simulink model "x2_Robot_Kin"  (R2024b)
settings: Solver=VariableStepAuto  StartTime=0.0  StopTime=inf  RelTol=1e-3  EnableMultiTasking=on
libraries: vrlib x7, simulink x6
settings Model: Creator=jorgemartins  LastModifiedBy=pinto
settings SolverCC: AlgebraicLoopSolver=TrustRegion
settings DataIOCC: LimitDataPoints=on  ReturnWorkspaceOutputs=off
settings OptimizationCC: LifeSpan=inf
settings DebuggingCC: UnconnectedInputMsg=warning  UnconnectedOutputMsg=warning  UnconnectedLineMsg=warning  AllowSymbolicDim=off  SFUnexpectedBacktrackingDiag=warning  SFNoUnconditionalDefaultTransitionDiag=warning  SFExecutionAtInitializationDiag=none  ArithmeticOperatorsInVariantConditions=warning
settings ModelReferenceCC: EnableRefExpFcnMdlSchedulingChecks=on  PropagateSignalLabelsOutOfModel=off
settings SFSimCC: SimUseLocalCustomCode=off  CustomCodeUndefinedFunction=UseInterfaceOnly
settings RTWCC: RTWUseLocalCustomCode=off  GPUComputeCapability=3.5
settings CodeAppCC: StateflowObjectComments=on
settings GRTTargetCC: TargetLangStandard=C89/C90 (ANSI)
settings ConfigComp: CovMetricSettings=dw  CovSaveCumulativeToWorkspaceVar=on  CovSaveSingleToWorkspaceVar=on  CovExternalEMLEnable=off

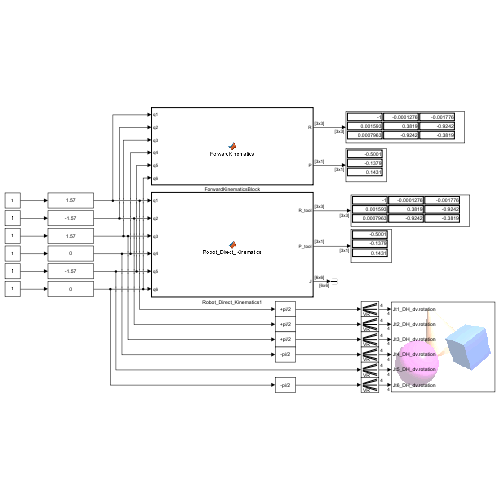
[thumbnail: Simulink's stored preview of the top-level diagram]
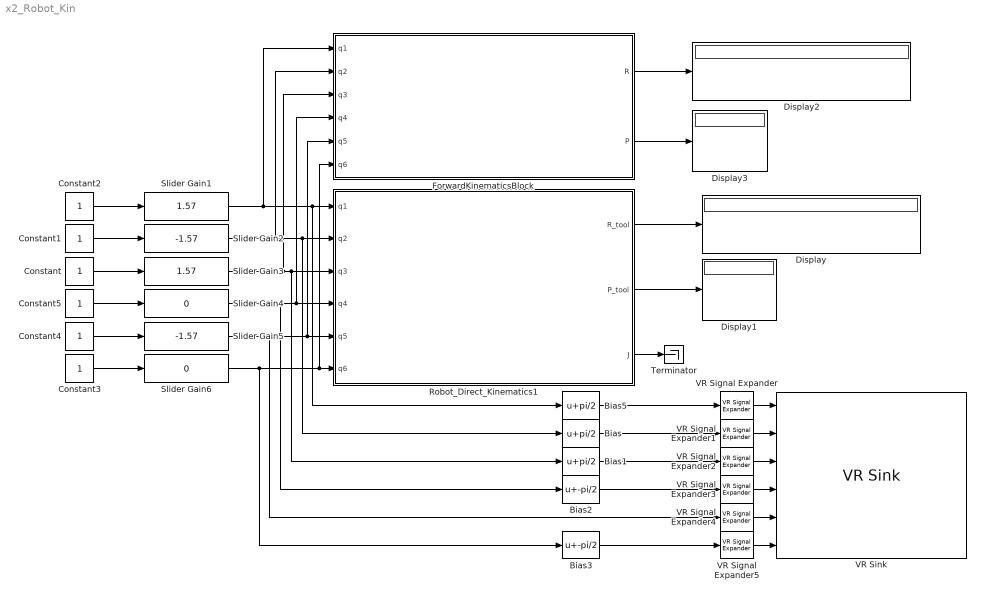
== system x2_Robot_Kin ==
  Bias : Bias  Bias=pi/2  SaturateOnIntegerOverflow=off
  Bias1 : Bias  Bias=pi/2  SaturateOnIntegerOverflow=off
  Bias2 : Bias  Bias=-pi/2  SaturateOnIntegerOverflow=off
  Bias3 : Bias  Bias=-pi/2  SaturateOnIntegerOverflow=off
  Bias5 : Bias  Bias=pi/2  SaturateOnIntegerOverflow=off
  Constant{,1..5} (6 alike) : Constant
  Display{,1..3} (4 alike) : Display
  ForwardKinematicsBlock : MATLAB Function  TreatAsAtomicUnit=on
  Robot_Direct_Kinematics1 : MATLAB Function  TreatAsAtomicUnit=on
  Slider Gain1 : simulink/Math Operations/Slider Gain  gain=1.57  low=-3.14  high=3.14
  Slider Gain2 : simulink/Math Operations/Slider Gain  gain=-1.57  low=-3.14  high=3.14
  Slider Gain3 : simulink/Math Operations/Slider Gain  gain=1.57  low=-3.14  high=3.14
  Slider Gain4 : simulink/Math Operations/Slider Gain  gain=0  low=-3.14  high=3.14
  Slider Gain5 : simulink/Math Operations/Slider Gain  gain=-1.57  low=-3.14  high=3.14
  Slider Gain6 : simulink/Math Operations/Slider Gain  gain=0  low=-3.14  high=3.14
  Terminator : Terminator
  VR Signal Expander{,1..5} (6 alike) : vrlib/VR Signal Expander  outwidth=4  outidx=[4]
  VR Sink : vrlib/VR Sink  InstantiateOnLoad=on  SampleTime=0.1  ViewEnable=on  RemoteChange=off  RemoteView=off  FieldsWritten=Jt1_DH_dv.rotation.4.1.1.double#Jt2_DH_dv.rotation.4.1.1.double#Jt3_DH_dv.rotation.4.1.1.double#Jt4_DH_dv.rotation.4.1.1.double#Jt5_DH_dv.rotation.4.1.1.double#Jt6_DH_dv.rotation.4.1.1.double  WorldFileName=vrrobot.wrl  WorldDescription=D-H Reference Frames for Virtual Reality Robot  AutoView=off  VideoDimensions=[]  AllowVariableSize=off
  wires:
  Robot_Direct_Kinematics1/1(R_tool) -> Display/1
  Robot_Direct_Kinematics1/2(P_tool) -> Display1/1
  Constant/1 -> Slider Gain3/1
  Slider Gain3/1 -> ForwardKinematicsBlock/3(q3), Robot_Direct_Kinematics1/3(q3), Bias1/1
  Constant2/1 -> Slider Gain1/1
  Slider Gain1/1 -> ForwardKinematicsBlock/1(q1), Robot_Direct_Kinematics1/1(q1), Bias5/1
  Constant1/1 -> Slider Gain2/1
  Slider Gain2/1 -> ForwardKinematicsBlock/2(q2), Robot_Direct_Kinematics1/2(q2), Bias/1
  Bias/1 -> VR Signal Expander1/1
  Bias1/1 -> VR Signal Expander2/1
  Constant4/1 -> Slider Gain5/1
  Slider Gain6/1 -> Robot_Direct_Kinematics1/6(q6), ForwardKinematicsBlock/6(q6), Bias3/1
  Constant3/1 -> Slider Gain6/1
  Slider Gain4/1 -> Robot_Direct_Kinematics1/4(q4), ForwardKinematicsBlock/4(q4), Bias2/1
  Constant5/1 -> Slider Gain4/1
  Bias3/1 -> VR Signal Expander5/1
  Slider Gain5/1 -> Robot_Direct_Kinematics1/5(q5), ForwardKinematicsBlock/5(q5), VR Signal Expander4/1
  Bias2/1 -> VR Signal Expander3/1
  Bias5/1 -> VR Signal Expander/1
  VR Signal Expander/1 -> VR Sink/1
  VR Signal Expander1/1 -> VR Sink/2
  VR Signal Expander2/1 -> VR Sink/3
  VR Signal Expander3/1 -> VR Sink/4
  VR Signal Expander4/1 -> VR Sink/5
  VR Signal Expander5/1 -> VR Sink/6
  ForwardKinematicsBlock/2(P) -> Display3/1
  ForwardKinematicsBlock/1(R) -> Display2/1
  Robot_Direct_Kinematics1/3(J) -> Terminator/1

== matlab function x2_Robot_Kin/ForwardKinematicsBlock ==
  data: q1 input; R output; q2 input; q3 input; q4 input; q5 input; q6 input; P output
function [R, P] = ForwardKinematics(q1, q2, q3, q4, q5, q6)

DH = [ 0     q1  0     pi/2      pi/2;
       0     q2  0    -pi/2      pi/2;
       0.4   q3  0     pi/2      pi/2;
       0     q4  0.1   pi/2     -pi/2;
       0.5   q5  0    -pi/2      0;
       0.1   q6  0     pi/2-pi/8 -pi/2;
       0.15  0   0     0         0 ];

T = eye(4);

for i = 1:size(DH,1)
    d = DH(i,1);
    theta = DH(i,2) + DH(i,5);
    a = DH(i,3);
    alpha = DH(i,4);

    A = [ cos(theta), -sin(theta)*cos(alpha),  sin(theta)*sin(alpha), a*cos(theta);
          sin(theta),  cos(theta)*cos(alpha), -cos(theta)*sin(alpha), a*sin(theta);
          0,           sin(alpha),             cos(alpha),            d;
          0,           0,                      0,                     1 ];

    T = T * A;
end

R = T(1:3, 1:3);
P = T(1:3, 4);

== matlab function x2_Robot_Kin/Robot_Direct_Kinematics1 ==
  data: q1 input; R_tool output; q2 input; q3 input; q4 input; q5 input; q6 input; P_tool output; J output
function [R_tool,P_tool,J] = Robot_Direct_Kinematics(q1,q2,q3,q4,q5,q6)
%#codegen

%    This function was generated by the Symbolic Math Toolbox version 24.2.
%    22-May-2025 17:53:28

% q1 = complex(q1);  % if required to enforce complex operations
% q2 = complex(q2);  % if required to enforce complex operations
% q3 = complex(q3);  % if required to enforce complex operations
% q4 = complex(q4);  % if required to enforce complex operations
% q5 = complex(q5);  % if required to enforce complex operations
% q6 = complex(q6);  % if required to enforce complex operations
et1 = cos(q5).*sin(q1).*sin(q3).*sqrt(sqrt(2.0)+2.0).*(-1.0./2.0)-(cos(q1).*cos(q2).*sin(q4).*sin(q6).*sqrt(-sqrt(2.0)+2.0))./2.0-(cos(q3).*cos(q4).*sin(q1).*sin(q6).*sqrt(-sqrt(2.0)+2.0))./2.0-(cos(q6).*sin(q1).*sin(q3).*sin(q5).*sqrt(-sqrt(2.0)+2.0))./2.0-(cos(q1).*cos(q3).*cos(q5).*sin(q2).*sqrt(sqrt(2.0)+2.0))./2.0-(cos(q1).*cos(q2).*cos(q4).*sin(q5).*sqrt(sqrt(2.0)+2.0))./2.0+(cos(q3).*sin(q1).*sin(q4).*sin(q5).*sqrt(sqrt(2.0)+2.0))./2.0;
et2 = (cos(q1).*cos(q2).*cos(q4).*cos(q5).*cos(q6).*sqrt(-sqrt(2.0)+2.0))./2.0-(cos(q1).*cos(q3).*cos(q6).*sin(q2).*sin(q5).*sqrt(-sqrt(2.0)+2.0))./2.0-(cos(q3).*cos(q5).*cos(q6).*sin(q1).*sin(q4).*sqrt(-sqrt(2.0)+2.0))./2.0+(cos(q1).*cos(q4).*sin(q2).*sin(q3).*sin(q6).*sqrt(-sqrt(2.0)+2.0))./2.0-(cos(q1).*sin(q2).*sin(q3).*sin(q4).*sin(q5).*sqrt(sqrt(2.0)+2.0))./2.0+(cos(q1).*cos(q5).*cos(q6).*sin(q2).*sin(q3).*sin(q4).*sqrt(-sqrt(2.0)+2.0))./2.0;
et3 = cos(q1).*cos(q5).*sin(q3).*sqrt(sqrt(2.0)+2.0).*(-1.0./2.0)-(cos(q1).*cos(q3).*cos(q4).*sin(q6).*sqrt(-sqrt(2.0)+2.0))./2.0-(cos(q1).*cos(q6).*sin(q3).*sin(q5).*sqrt(-sqrt(2.0)+2.0))./2.0+(cos(q2).*sin(q1).*sin(q4).*sin(q6).*sqrt(-sqrt(2.0)+2.0))./2.0+(cos(q3).*cos(q5).*sin(q1).*sin(q2).*sqrt(sqrt(2.0)+2.0))./2.0+(cos(q2).*cos(q4).*sin(q1).*sin(q5).*sqrt(sqrt(2.0)+2.0))./2.0+(cos(q1).*cos(q3).*sin(q4).*sin(q5).*sqrt(sqrt(2.0)+2.0))./2.0-(cos(q2).*cos(q4).*cos(q5).*cos(q6).*sin(q1).*sqrt(-sqrt(2.0)+2.0))./2.0;
et4 = cos(q1).*cos(q3).*cos(q5).*cos(q6).*sin(q4).*sqrt(-sqrt(2.0)+2.0).*(-1.0./2.0)+(cos(q3).*cos(q6).*sin(q1).*sin(q2).*sin(q5).*sqrt(-sqrt(2.0)+2.0))./2.0-(cos(q4).*sin(q1).*sin(q2).*sin(q3).*sin(q6).*sqrt(-sqrt(2.0)+2.0))./2.0+(sin(q1).*sin(q2).*sin(q3).*sin(q4).*sin(q5).*sqrt(sqrt(2.0)+2.0))./2.0-(cos(q5).*cos(q6).*sin(q1).*sin(q2).*sin(q3).*sin(q4).*sqrt(-sqrt(2.0)+2.0))./2.0;
et5 = cos(q5).*sin(q1).*sin(q3).*sqrt(-sqrt(2.0)+2.0).*(-1.0./2.0)-(cos(q1).*cos(q3).*cos(q5).*sin(q2).*sqrt(-sqrt(2.0)+2.0))./2.0-(cos(q1).*cos(q2).*cos(q4).*sin(q5).*sqrt(-sqrt(2.0)+2.0))./2.0+(cos(q3).*sin(q1).*sin(q4).*sin(q5).*sqrt(-sqrt(2.0)+2.0))./2.0+(cos(q1).*cos(q2).*sin(q4).*sin(q6).*sqrt(sqrt(2.0)+2.0))./2.0+(cos(q3).*cos(q4).*sin(q1).*sin(q6).*sqrt(sqrt(2.0)+2.0))./2.0+(cos(q6).*sin(q1).*sin(q3).*sin(q5).*sqrt(sqrt(2.0)+2.0))./2.0;
et6 = cos(q1).*sin(q2).*sin(q3).*sin(q4).*sin(q5).*sqrt(-sqrt(2.0)+2.0).*(-1.0./2.0)-(cos(q1).*cos(q2).*cos(q4).*cos(q5).*cos(q6).*sqrt(sqrt(2.0)+2.0))./2.0+(cos(q1).*cos(q3).*cos(q6).*sin(q2).*sin(q5).*sqrt(sqrt(2.0)+2.0))./2.0+(cos(q3).*cos(q5).*cos(q6).*sin(q1).*sin(q4).*sqrt(sqrt(2.0)+2.0))./2.0-(cos(q1).*cos(q4).*sin(q2).*sin(q3).*sin(q6).*sqrt(sqrt(2.0)+2.0))./2.0-(cos(q1).*cos(q5).*cos(q6).*sin(q2).*sin(q3).*sin(q4).*sqrt(sqrt(2.0)+2.0))./2.0;
et7 = cos(q1).*cos(q5).*sin(q3).*sqrt(-sqrt(2.0)+2.0).*(-1.0./2.0)+(cos(q3).*cos(q5).*sin(q1).*sin(q2).*sqrt(-sqrt(2.0)+2.0))./2.0+(cos(q2).*cos(q4).*sin(q1).*sin(q5).*sqrt(-sqrt(2.0)+2.0))./2.0+(cos(q1).*cos(q3).*sin(q4).*sin(q5).*sqrt(-sqrt(2.0)+2.0))./2.0+(cos(q1).*cos(q3).*cos(q4).*sin(q6).*sqrt(sqrt(2.0)+2.0))./2.0+(cos(q1).*cos(q6).*sin(q3).*sin(q5).*sqrt(sqrt(2.0)+2.0))./2.0-(cos(q2).*sin(q1).*sin(q4).*sin(q6).*sqrt(sqrt(2.0)+2.0))./2.0;
et8 = (sin(q1).*sin(q2).*sin(q3).*sin(q4).*sin(q5).*sqrt(-sqrt(2.0)+2.0))./2.0+(cos(q2).*cos(q4).*cos(q5).*cos(q6).*sin(q1).*sqrt(sqrt(2.0)+2.0))./2.0+(cos(q1).*cos(q3).*cos(q5).*cos(q6).*sin(q4).*sqrt(sqrt(2.0)+2.0))./2.0-(cos(q3).*cos(q6).*sin(q1).*sin(q2).*sin(q5).*sqrt(sqrt(2.0)+2.0))./2.0+(cos(q4).*sin(q1).*sin(q2).*sin(q3).*sin(q6).*sqrt(sqrt(2.0)+2.0))./2.0+(cos(q5).*cos(q6).*sin(q1).*sin(q2).*sin(q3).*sin(q4).*sqrt(sqrt(2.0)+2.0))./2.0;
mt1 = [cos(q1).*cos(q3).*cos(q4).*cos(q6)-cos(q2).*cos(q6).*sin(q1).*sin(q4)-cos(q1).*sin(q3).*sin(q5).*sin(q6)-cos(q2).*cos(q4).*cos(q5).*sin(q1).*sin(q6)-cos(q1).*cos(q3).*cos(q5).*sin(q4).*sin(q6)+cos(q4).*cos(q6).*sin(q1).*sin(q2).*sin(q3)+cos(q3).*sin(q1).*sin(q2).*sin(q5).*sin(q6)-cos(q5).*sin(q1).*sin(q2).*sin(q3).*sin(q4).*sin(q6),cos(q1).*cos(q2).*cos(q6).*sin(q4)+cos(q3).*cos(q4).*cos(q6).*sin(q1)-sin(q1).*sin(q3).*sin(q5).*sin(q6)+cos(q1).*cos(q2).*cos(q4).*cos(q5).*sin(q6)-cos(q1).*cos(q4).*cos(q6).*sin(q2).*sin(q3)-cos(q1).*cos(q3).*sin(q2).*sin(q5).*sin(q6)-cos(q3).*cos(q5).*sin(q1).*sin(q4).*sin(q6)+cos(q1).*cos(q5).*sin(q2).*sin(q3).*sin(q4).*sin(q6)];
mt2 = [cos(q6).*sin(q2).*sin(q4)+cos(q2).*cos(q4).*cos(q6).*sin(q3)+cos(q2).*cos(q3).*sin(q5).*sin(q6)+cos(q4).*cos(q5).*sin(q2).*sin(q6)-cos(q2).*cos(q5).*sin(q3).*sin(q4).*sin(q6),et3+et4,et1+et2];
mt3 = [cos(q4).*sin(q2).*sin(q5).*sqrt(sqrt(2.0)+2.0).*(-1.0./2.0)-(sin(q2).*sin(q4).*sin(q6).*sqrt(-sqrt(2.0)+2.0))./2.0+(cos(q2).*cos(q3).*cos(q5).*sqrt(sqrt(2.0)+2.0))./2.0+(cos(q2).*cos(q3).*cos(q6).*sin(q5).*sqrt(-sqrt(2.0)+2.0))./2.0+(cos(q4).*cos(q5).*cos(q6).*sin(q2).*sqrt(-sqrt(2.0)+2.0))./2.0-(cos(q2).*cos(q4).*sin(q3).*sin(q6).*sqrt(-sqrt(2.0)+2.0))./2.0+(cos(q2).*sin(q3).*sin(q4).*sin(q5).*sqrt(sqrt(2.0)+2.0))./2.0-(cos(q2).*cos(q5).*cos(q6).*sin(q3).*sin(q4).*sqrt(-sqrt(2.0)+2.0))./2.0];
mt4 = [et7+et8,et5+et6,(sin(q2).*sin(q4).*sin(q6).*sqrt(sqrt(2.0)+2.0))./2.0+(cos(q2).*cos(q3).*cos(q5).*sqrt(-sqrt(2.0)+2.0))./2.0-(cos(q4).*sin(q2).*sin(q5).*sqrt(-sqrt(2.0)+2.0))./2.0+(cos(q2).*sin(q3).*sin(q4).*sin(q5).*sqrt(-sqrt(2.0)+2.0))./2.0-(cos(q2).*cos(q3).*cos(q6).*sin(q5).*sqrt(sqrt(2.0)+2.0))./2.0-(cos(q4).*cos(q5).*cos(q6).*sin(q2).*sqrt(sqrt(2.0)+2.0))./2.0+(cos(q2).*cos(q4).*sin(q3).*sin(q6).*sqrt(sqrt(2.0)+2.0))./2.0+(cos(q2).*cos(q5).*cos(q6).*sin(q3).*sin(q4).*sqrt(sqrt(2.0)+2.0))./2.0];
R_tool = reshape([mt1,mt2,mt3,mt4],3,3);
if nargout > 1
    et9 = sin(q2).*(-2.0./5.0)+(cos(q4).*sin(q2))./1.0e+1+(sin(q2).*sin(q4))./2.0+(cos(q2).*cos(q3).*cos(q5))./1.0e+1+(cos(q2).*cos(q4).*sin(q3))./2.0-(cos(q2).*sin(q3).*sin(q4))./1.0e+1-(cos(q4).*sin(q2).*sin(q5))./1.0e+1+sin(q2).*sin(q4).*sin(q6).*sqrt(sqrt(2.0)+2.0).*(3.0./4.0e+1)+cos(q2).*cos(q3).*cos(q5).*sqrt(-sqrt(2.0)+2.0).*(3.0./4.0e+1)-cos(q4).*sin(q2).*sin(q5).*sqrt(-sqrt(2.0)+2.0).*(3.0./4.0e+1)+(cos(q2).*sin(q3).*sin(q4).*sin(q5))./1.0e+1+cos(q2).*sin(q3).*sin(q4).*sin(q5).*sqrt(-sqrt(2.0)+2.0).*(3.0./4.0e+1);
    et10 = cos(q2).*cos(q3).*cos(q6).*sin(q5).*sqrt(sqrt(2.0)+2.0).*(-3.0./4.0e+1)-cos(q4).*cos(q5).*cos(q6).*sin(q2).*sqrt(sqrt(2.0)+2.0).*(3.0./4.0e+1)+cos(q2).*cos(q4).*sin(q3).*sin(q6).*sqrt(sqrt(2.0)+2.0).*(3.0./4.0e+1)+cos(q2).*cos(q5).*cos(q6).*sin(q3).*sin(q4).*sqrt(sqrt(2.0)+2.0).*(3.0./4.0e+1);
    et11 = cos(q1).*cos(q2).*(-2.0./5.0)+(cos(q1).*cos(q2).*cos(q4))./1.0e+1+(cos(q1).*cos(q2).*sin(q4))./2.0+(cos(q3).*cos(q4).*sin(q1))./2.0-(cos(q3).*sin(q1).*sin(q4))./1.0e+1-(cos(q5).*sin(q1).*sin(q3))./1.0e+1-cos(q5).*sin(q1).*sin(q3).*sqrt(-sqrt(2.0)+2.0).*(3.0./4.0e+1)-(cos(q1).*cos(q3).*cos(q5).*sin(q2))./1.0e+1-(cos(q1).*cos(q2).*cos(q4).*sin(q5))./1.0e+1-(cos(q1).*cos(q4).*sin(q2).*sin(q3))./2.0+(cos(q1).*sin(q2).*sin(q3).*sin(q4))./1.0e+1+(cos(q3).*sin(q1).*sin(q4).*sin(q5))./1.0e+1-cos(q1).*cos(q3).*cos(q5).*sin(q2).*sqrt(-sqrt(2.0)+2.0).*(3.0./4.0e+1);
    et12 = cos(q1).*cos(q2).*cos(q4).*sin(q5).*sqrt(-sqrt(2.0)+2.0).*(-3.0./4.0e+1)+cos(q3).*sin(q1).*sin(q4).*sin(q5).*sqrt(-sqrt(2.0)+2.0).*(3.0./4.0e+1)-(cos(q1).*sin(q2).*sin(q3).*sin(q4).*sin(q5))./1.0e+1+cos(q1).*cos(q2).*sin(q4).*sin(q6).*sqrt(sqrt(2.0)+2.0).*(3.0./4.0e+1)+cos(q3).*cos(q4).*sin(q1).*sin(q6).*sqrt(sqrt(2.0)+2.0).*(3.0./4.0e+1)+cos(q6).*sin(q1).*sin(q3).*sin(q5).*sqrt(sqrt(2.0)+2.0).*(3.0./4.0e+1)-cos(q1).*sin(q2).*sin(q3).*sin(q4).*sin(q5).*sqrt(-sqrt(2.0)+2.0).*(3.0./4.0e+1)-cos(q1).*cos(q2).*cos(q4).*cos(q5).*cos(q6).*sqrt(sqrt(2.0)+2.0).*(3.0./4.0e+1);
    et13 = cos(q1).*cos(q3).*cos(q6).*sin(q2).*sin(q5).*sqrt(sqrt(2.0)+2.0).*(3.0./4.0e+1)+cos(q3).*cos(q5).*cos(q6).*sin(q1).*sin(q4).*sqrt(sqrt(2.0)+2.0).*(3.0./4.0e+1)-cos(q1).*cos(q4).*sin(q2).*sin(q3).*sin(q6).*sqrt(sqrt(2.0)+2.0).*(3.0./4.0e+1)-cos(q1).*cos(q5).*cos(q6).*sin(q2).*sin(q3).*sin(q4).*sqrt(sqrt(2.0)+2.0).*(3.0./4.0e+1);
    et14 = cos(q2).*sin(q1).*(2.0./5.0)+(cos(q1).*cos(q3).*cos(q4))./2.0-(cos(q2).*cos(q4).*sin(q1))./1.0e+1-(cos(q1).*cos(q3).*sin(q4))./1.0e+1-(cos(q1).*cos(q5).*sin(q3))./1.0e+1-(cos(q2).*sin(q1).*sin(q4))./2.0-cos(q1).*cos(q5).*sin(q3).*sqrt(-sqrt(2.0)+2.0).*(3.0./4.0e+1)+(cos(q3).*cos(q5).*sin(q1).*sin(q2))./1.0e+1+(cos(q2).*cos(q4).*sin(q1).*sin(q5))./1.0e+1+(cos(q1).*cos(q3).*sin(q4).*sin(q5))./1.0e+1+(cos(q4).*sin(q1).*sin(q2).*sin(q3))./2.0-(sin(q1).*sin(q2).*sin(q3).*sin(q4))./1.0e+1+cos(q3).*cos(q5).*sin(q1).*sin(q2).*sqrt(-sqrt(2.0)+2.0).*(3.0./4.0e+1);
    et15 = cos(q2).*cos(q4).*sin(q1).*sin(q5).*sqrt(-sqrt(2.0)+2.0).*(3.0./4.0e+1)+cos(q1).*cos(q3).*sin(q4).*sin(q5).*sqrt(-sqrt(2.0)+2.0).*(3.0./4.0e+1)+(sin(q1).*sin(q2).*sin(q3).*sin(q4).*sin(q5))./1.0e+1+cos(q1).*cos(q3).*cos(q4).*sin(q6).*sqrt(sqrt(2.0)+2.0).*(3.0./4.0e+1)+cos(q1).*cos(q6).*sin(q3).*sin(q5).*sqrt(sqrt(2.0)+2.0).*(3.0./4.0e+1)-cos(q2).*sin(q1).*sin(q4).*sin(q6).*sqrt(sqrt(2.0)+2.0).*(3.0./4.0e+1)+sin(q1).*sin(q2).*sin(q3).*sin(q4).*sin(q5).*sqrt(-sqrt(2.0)+2.0).*(3.0./4.0e+1)+cos(q2).*cos(q4).*cos(q5).*cos(q6).*sin(q1).*sqrt(sqrt(2.0)+2.0).*(3.0./4.0e+1);
    et16 = cos(q1).*cos(q3).*cos(q5).*cos(q6).*sin(q4).*sqrt(sqrt(2.0)+2.0).*(3.0./4.0e+1)-cos(q3).*cos(q6).*sin(q1).*sin(q2).*sin(q5).*sqrt(sqrt(2.0)+2.0).*(3.0./4.0e+1)+cos(q4).*sin(q1).*sin(q2).*sin(q3).*sin(q6).*sqrt(sqrt(2.0)+2.0).*(3.0./4.0e+1)+cos(q5).*cos(q6).*sin(q1).*sin(q2).*sin(q3).*sin(q4).*sqrt(sqrt(2.0)+2.0).*(3.0./4.0e+1);
    P_tool = [et14+et15+et16;et11+et12+et13;et9+et10];
end
if nargout > 2
    et17 = cos(q2).*sin(q1).*(2.0./5.0)+(cos(q1).*cos(q3).*cos(q4))./2.0-(cos(q2).*cos(q4).*sin(q1))./1.0e+1-(cos(q1).*cos(q3).*sin(q4))./1.0e+1-(cos(q1).*cos(q5).*sin(q3))./1.0e+1-(cos(q2).*sin(q1).*sin(q4))./2.0-cos(q1).*cos(q5).*sin(q3).*sqrt(-sqrt(2.0)+2.0).*(3.0./4.0e+1)+(cos(q3).*cos(q5).*sin(q1).*sin(q2))./1.0e+1+(cos(q2).*cos(q4).*sin(q1).*sin(q5))./1.0e+1+(cos(q1).*cos(q3).*sin(q4).*sin(q5))./1.0e+1+(cos(q4).*sin(q1).*sin(q2).*sin(q3))./2.0-(sin(q1).*sin(q2).*sin(q3).*sin(q4))./1.0e+1+cos(q3).*cos(q5).*sin(q1).*sin(q2).*sqrt(-sqrt(2.0)+2.0).*(3.0./4.0e+1);
    et18 = cos(q2).*cos(q4).*sin(q1).*sin(q5).*sqrt(-sqrt(2.0)+2.0).*(3.0./4.0e+1)+cos(q1).*cos(q3).*sin(q4).*sin(q5).*sqrt(-sqrt(2.0)+2.0).*(3.0./4.0e+1)+(sin(q1).*sin(q2).*sin(q3).*sin(q4).*sin(q5))./1.0e+1+cos(q1).*cos(q3).*cos(q4).*sin(q6).*sqrt(sqrt(2.0)+2.0).*(3.0./4.0e+1)+cos(q1).*cos(q6).*sin(q3).*sin(q5).*sqrt(sqrt(2.0)+2.0).*(3.0./4.0e+1)-cos(q2).*sin(q1).*sin(q4).*sin(q6).*sqrt(sqrt(2.0)+2.0).*(3.0./4.0e+1)+sin(q1).*sin(q2).*sin(q3).*sin(q4).*sin(q5).*sqrt(-sqrt(2.0)+2.0).*(3.0./4.0e+1)+cos(q2).*cos(q4).*cos(q5).*cos(q6).*sin(q1).*sqrt(sqrt(2.0)+2.0).*(3.0./4.0e+1);
    et19 = cos(q1).*cos(q3).*cos(q5).*cos(q6).*sin(q4).*sqrt(sqrt(2.0)+2.0).*(3.0./4.0e+1)-cos(q3).*cos(q6).*sin(q1).*sin(q2).*sin(q5).*sqrt(sqrt(2.0)+2.0).*(3.0./4.0e+1)+cos(q4).*sin(q1).*sin(q2).*sin(q3).*sin(q6).*sqrt(sqrt(2.0)+2.0).*(3.0./4.0e+1)+cos(q5).*cos(q6).*sin(q1).*sin(q2).*sin(q3).*sin(q4).*sqrt(sqrt(2.0)+2.0).*(3.0./4.0e+1);
    et20 = cos(q1).*cos(q2).*(2.0./5.0)-(cos(q1).*cos(q2).*cos(q4))./1.0e+1-(cos(q1).*cos(q2).*sin(q4))./2.0-(cos(q3).*cos(q4).*sin(q1))./2.0+(cos(q3).*sin(q1).*sin(q4))./1.0e+1+(cos(q5).*sin(q1).*sin(q3))./1.0e+1+cos(q5).*sin(q1).*sin(q3).*sqrt(-sqrt(2.0)+2.0).*(3.0./4.0e+1)+(cos(q1).*cos(q3).*cos(q5).*sin(q2))./1.0e+1+(cos(q1).*cos(q2).*cos(q4).*sin(q5))./1.0e+1+(cos(q1).*cos(q4).*sin(q2).*sin(q3))./2.0-(cos(q1).*sin(q2).*sin(q3).*sin(q4))./1.0e+1-(cos(q3).*sin(q1).*sin(q4).*sin(q5))./1.0e+1+cos(q1).*cos(q3).*cos(q5).*sin(q2).*sqrt(-sqrt(2.0)+2.0).*(3.0./4.0e+1);
    et21 = cos(q1).*cos(q2).*cos(q4).*sin(q5).*sqrt(-sqrt(2.0)+2.0).*(3.0./4.0e+1)-cos(q3).*sin(q1).*sin(q4).*sin(q5).*sqrt(-sqrt(2.0)+2.0).*(3.0./4.0e+1)+(cos(q1).*sin(q2).*sin(q3).*sin(q4).*sin(q5))./1.0e+1-cos(q1).*cos(q2).*sin(q4).*sin(q6).*sqrt(sqrt(2.0)+2.0).*(3.0./4.0e+1)-cos(q3).*cos(q4).*sin(q1).*sin(q6).*sqrt(sqrt(2.0)+2.0).*(3.0./4.0e+1)-cos(q6).*sin(q1).*sin(q3).*sin(q5).*sqrt(sqrt(2.0)+2.0).*(3.0./4.0e+1)+cos(q1).*sin(q2).*sin(q3).*sin(q4).*sin(q5).*sqrt(-sqrt(2.0)+2.0).*(3.0./4.0e+1)+cos(q1).*cos(q2).*cos(q4).*cos(q5).*cos(q6).*sqrt(sqrt(2.0)+2.0).*(3.0./4.0e+1);
    et22 = cos(q1).*cos(q3).*cos(q6).*sin(q2).*sin(q5).*sqrt(sqrt(2.0)+2.0).*(-3.0./4.0e+1)-cos(q3).*cos(q5).*cos(q6).*sin(q1).*sin(q4).*sqrt(sqrt(2.0)+2.0).*(3.0./4.0e+1)+cos(q1).*cos(q4).*sin(q2).*sin(q3).*sin(q6).*sqrt(sqrt(2.0)+2.0).*(3.0./4.0e+1)+cos(q1).*cos(q5).*cos(q6).*sin(q2).*sin(q3).*sin(q4).*sqrt(sqrt(2.0)+2.0).*(3.0./4.0e+1);
    et23 = cos(q2).*(-2.0./5.0)+(cos(q2).*cos(q4))./1.0e+1+(cos(q2).*sin(q4))./2.0+(sin(q2).*sin(q3).*sin(q4))./1.0e+1-(cos(q3).*cos(q5).*sin(q2))./1.0e+1-(cos(q2).*cos(q4).*sin(q5))./1.0e+1-(cos(q4).*sin(q2).*sin(q3))./2.0+cos(q2).*sin(q4).*sin(q6).*sqrt(sqrt(2.0)+2.0).*(3.0./4.0e+1)-cos(q3).*cos(q5).*sin(q2).*sqrt(-sqrt(2.0)+2.0).*(3.0./4.0e+1)-cos(q2).*cos(q4).*sin(q5).*sqrt(-sqrt(2.0)+2.0).*(3.0./4.0e+1)-(sin(q2).*sin(q3).*sin(q4).*sin(q5))./1.0e+1-sin(q2).*sin(q3).*sin(q4).*sin(q5).*sqrt(-sqrt(2.0)+2.0).*(3.0./4.0e+1);
    et24 = cos(q2).*cos(q4).*cos(q5).*cos(q6).*sqrt(sqrt(2.0)+2.0).*(-3.0./4.0e+1)+cos(q3).*cos(q6).*sin(q2).*sin(q5).*sqrt(sqrt(2.0)+2.0).*(3.0./4.0e+1)-cos(q4).*sin(q2).*sin(q3).*sin(q6).*sqrt(sqrt(2.0)+2.0).*(3.0./4.0e+1)-cos(q5).*cos(q6).*sin(q2).*sin(q3).*sin(q4).*sqrt(sqrt(2.0)+2.0).*(3.0./4.0e+1);
    et25 = sin(q2).*-1.6e+1+cos(q4).*sin(q2).*4.0+sin(q2).*sin(q4).*2.0e+1+cos(q2).*cos(q3).*cos(q5).*4.0+cos(q2).*cos(q4).*sin(q3).*2.0e+1-cos(q2).*sin(q3).*sin(q4).*4.0-cos(q4).*sin(q2).*sin(q5).*4.0+sin(q2).*sin(q4).*sin(q6).*sqrt(sqrt(2.0)+2.0).*3.0+cos(q2).*cos(q3).*cos(q5).*sqrt(-sqrt(2.0)+2.0).*3.0-cos(q4).*sin(q2).*sin(q5).*sqrt(-sqrt(2.0)+2.0).*3.0+cos(q2).*sin(q3).*sin(q4).*sin(q5).*4.0+cos(q2).*sin(q3).*sin(q4).*sin(q5).*sqrt(-sqrt(2.0)+2.0).*3.0-cos(q2).*cos(q3).*cos(q6).*sin(q5).*sqrt(sqrt(2.0)+2.0).*3.0-cos(q4).*cos(q5).*cos(q6).*sin(q2).*sqrt(sqrt(2.0)+2.0).*3.0;
    et26 = cos(q2).*cos(q4).*sin(q3).*sin(q6).*sqrt(sqrt(2.0)+2.0).*3.0+cos(q2).*cos(q5).*cos(q6).*sin(q3).*sin(q4).*sqrt(sqrt(2.0)+2.0).*3.0;
    et27 = sin(q2).*-1.6e+1+cos(q4).*sin(q2).*4.0+sin(q2).*sin(q4).*2.0e+1+cos(q2).*cos(q3).*cos(q5).*4.0+cos(q2).*cos(q4).*sin(q3).*2.0e+1-cos(q2).*sin(q3).*sin(q4).*4.0-cos(q4).*sin(q2).*sin(q5).*4.0+sin(q2).*sin(q4).*sin(q6).*sqrt(sqrt(2.0)+2.0).*3.0+cos(q2).*cos(q3).*cos(q5).*sqrt(-sqrt(2.0)+2.0).*3.0-cos(q4).*sin(q2).*sin(q5).*sqrt(-sqrt(2.0)+2.0).*3.0+cos(q2).*sin(q3).*sin(q4).*sin(q5).*4.0+cos(q2).*sin(q3).*sin(q4).*sin(q5).*sqrt(-sqrt(2.0)+2.0).*3.0-cos(q2).*cos(q3).*cos(q6).*sin(q5).*sqrt(sqrt(2.0)+2.0).*3.0-cos(q4).*cos(q5).*cos(q6).*sin(q2).*sqrt(sqrt(2.0)+2.0).*3.0;
    et28 = cos(q2).*cos(q4).*sin(q3).*sin(q6).*sqrt(sqrt(2.0)+2.0).*3.0+cos(q2).*cos(q5).*cos(q6).*sin(q3).*sin(q4).*sqrt(sqrt(2.0)+2.0).*3.0;
    et29 = (sin(q1).*sin(q3).*sin(q4))./1.0e+1-(cos(q3).*cos(q5).*sin(q1))./1.0e+1-(cos(q4).*sin(q1).*sin(q3))./2.0-cos(q3).*cos(q5).*sin(q1).*sqrt(-sqrt(2.0)+2.0).*(3.0./4.0e+1)-(cos(q1).*cos(q3).*cos(q4).*sin(q2))./2.0+(cos(q1).*cos(q3).*sin(q2).*sin(q4))./1.0e+1+(cos(q1).*cos(q5).*sin(q2).*sin(q3))./1.0e+1-(sin(q1).*sin(q3).*sin(q4).*sin(q5))./1.0e+1+cos(q1).*cos(q5).*sin(q2).*sin(q3).*sqrt(-sqrt(2.0)+2.0).*(3.0./4.0e+1)-sin(q1).*sin(q3).*sin(q4).*sin(q5).*sqrt(-sqrt(2.0)+2.0).*(3.0./4.0e+1)-(cos(q1).*cos(q3).*sin(q2).*sin(q4).*sin(q5))./1.0e+1;
    et30 = cos(q3).*cos(q6).*sin(q1).*sin(q5).*sqrt(sqrt(2.0)+2.0).*(3.0./4.0e+1)-cos(q4).*sin(q1).*sin(q3).*sin(q6).*sqrt(sqrt(2.0)+2.0).*(3.0./4.0e+1)-cos(q1).*cos(q3).*sin(q2).*sin(q4).*sin(q5).*sqrt(-sqrt(2.0)+2.0).*(3.0./4.0e+1)-cos(q1).*cos(q3).*cos(q4).*sin(q2).*sin(q6).*sqrt(sqrt(2.0)+2.0).*(3.0./4.0e+1)-cos(q1).*cos(q6).*sin(q2).*sin(q3).*sin(q5).*sqrt(sqrt(2.0)+2.0).*(3.0./4.0e+1)-cos(q5).*cos(q6).*sin(q1).*sin(q3).*sin(q4).*sqrt(sqrt(2.0)+2.0).*(3.0./4.0e+1)-cos(q1).*cos(q3).*cos(q5).*cos(q6).*sin(q2).*sin(q4).*sqrt(sqrt(2.0)+2.0).*(3.0./4.0e+1);
    et31 = cos(q1).*cos(q3).*cos(q5).*(-1.0./1.0e+1)-(cos(q1).*cos(q4).*sin(q3))./2.0+(cos(q1).*sin(q3).*sin(q4))./1.0e+1-cos(q1).*cos(q3).*cos(q5).*sqrt(-sqrt(2.0)+2.0).*(3.0./4.0e+1)+(cos(q3).*cos(q4).*sin(q1).*sin(q2))./2.0-(cos(q3).*sin(q1).*sin(q2).*sin(q4))./1.0e+1-(cos(q5).*sin(q1).*sin(q2).*sin(q3))./1.0e+1-(cos(q1).*sin(q3).*sin(q4).*sin(q5))./1.0e+1-cos(q5).*sin(q1).*sin(q2).*sin(q3).*sqrt(-sqrt(2.0)+2.0).*(3.0./4.0e+1)-cos(q1).*sin(q3).*sin(q4).*sin(q5).*sqrt(-sqrt(2.0)+2.0).*(3.0./4.0e+1)+(cos(q3).*sin(q1).*sin(q2).*sin(q4).*sin(q5))./1.0e+1;
    et32 = cos(q1).*cos(q3).*cos(q6).*sin(q5).*sqrt(sqrt(2.0)+2.0).*(3.0./4.0e+1)-cos(q1).*cos(q4).*sin(q3).*sin(q6).*sqrt(sqrt(2.0)+2.0).*(3.0./4.0e+1)+cos(q3).*sin(q1).*sin(q2).*sin(q4).*sin(q5).*sqrt(-sqrt(2.0)+2.0).*(3.0./4.0e+1)-cos(q1).*cos(q5).*cos(q6).*sin(q3).*sin(q4).*sqrt(sqrt(2.0)+2.0).*(3.0./4.0e+1)+cos(q3).*cos(q4).*sin(q1).*sin(q2).*sin(q6).*sqrt(sqrt(2.0)+2.0).*(3.0./4.0e+1)+cos(q6).*sin(q1).*sin(q2).*sin(q3).*sin(q5).*sqrt(sqrt(2.0)+2.0).*(3.0./4.0e+1)+cos(q3).*cos(q5).*cos(q6).*sin(q1).*sin(q2).*sin(q4).*sqrt(sqrt(2.0)+2.0).*(3.0./4.0e+1);
    et33 = (cos(q4).*sin(q2))./2.0-(sin(q2).*sin(q4))./1.0e+1+(sin(q2).*sin(q4).*sin(q5))./1.0e+1-(cos(q2).*cos(q4).*sin(q3))./1.0e+1-(cos(q2).*sin(q3).*sin(q4))./2.0+cos(q4).*sin(q2).*sin(q6).*sqrt(sqrt(2.0)+2.0).*(3.0./4.0e+1)+sin(q2).*sin(q4).*sin(q5).*sqrt(-sqrt(2.0)+2.0).*(3.0./4.0e+1)+(cos(q2).*cos(q4).*sin(q3).*sin(q5))./1.0e+1+cos(q2).*cos(q4).*sin(q3).*sin(q5).*sqrt(-sqrt(2.0)+2.0).*(3.0./4.0e+1)+cos(q5).*cos(q6).*sin(q2).*sin(q4).*sqrt(sqrt(2.0)+2.0).*(3.0./4.0e+1)-cos(q2).*sin(q3).*sin(q4).*sin(q6).*sqrt(sqrt(2.0)+2.0).*(3.0./4.0e+1);
    et34 = cos(q2).*cos(q4).*cos(q5).*cos(q6).*sin(q3).*sqrt(sqrt(2.0)+2.0).*(3.0./4.0e+1);
    et35 = (cos(q1).*cos(q2).*cos(q4))./2.0-(cos(q1).*cos(q2).*sin(q4))./1.0e+1-(cos(q3).*cos(q4).*sin(q1))./1.0e+1-(cos(q3).*sin(q1).*sin(q4))./2.0+(cos(q1).*cos(q4).*sin(q2).*sin(q3))./1.0e+1+(cos(q1).*cos(q2).*sin(q4).*sin(q5))./1.0e+1+(cos(q3).*cos(q4).*sin(q1).*sin(q5))./1.0e+1+(cos(q1).*sin(q2).*sin(q3).*sin(q4))./2.0+cos(q1).*cos(q2).*sin(q4).*sin(q5).*sqrt(-sqrt(2.0)+2.0).*(3.0./4.0e+1)+cos(q3).*cos(q4).*sin(q1).*sin(q5).*sqrt(-sqrt(2.0)+2.0).*(3.0./4.0e+1)-(cos(q1).*cos(q4).*sin(q2).*sin(q3).*sin(q5))./1.0e+1+cos(q1).*cos(q2).*cos(q4).*sin(q6).*sqrt(sqrt(2.0)+2.0).*(3.0./4.0e+1);
    et36 = cos(q3).*sin(q1).*sin(q4).*sin(q6).*sqrt(sqrt(2.0)+2.0).*(-3.0./4.0e+1)-cos(q1).*cos(q4).*sin(q2).*sin(q3).*sin(q5).*sqrt(-sqrt(2.0)+2.0).*(3.0./4.0e+1)+cos(q1).*cos(q2).*cos(q5).*cos(q6).*sin(q4).*sqrt(sqrt(2.0)+2.0).*(3.0./4.0e+1)+cos(q3).*cos(q4).*cos(q5).*cos(q6).*sin(q1).*sqrt(sqrt(2.0)+2.0).*(3.0./4.0e+1)+cos(q1).*sin(q2).*sin(q3).*sin(q4).*sin(q6).*sqrt(sqrt(2.0)+2.0).*(3.0./4.0e+1)-cos(q1).*cos(q4).*cos(q5).*cos(q6).*sin(q2).*sin(q3).*sqrt(sqrt(2.0)+2.0).*(3.0./4.0e+1);
    et37 = cos(q1).*cos(q3).*cos(q4).*(-1.0./1.0e+1)-(cos(q2).*cos(q4).*sin(q1))./2.0-(cos(q1).*cos(q3).*sin(q4))./2.0+(cos(q2).*sin(q1).*sin(q4))./1.0e+1+(cos(q1).*cos(q3).*cos(q4).*sin(q5))./1.0e+1-(cos(q4).*sin(q1).*sin(q2).*sin(q3))./1.0e+1-(cos(q2).*sin(q1).*sin(q4).*sin(q5))./1.0e+1-(sin(q1).*sin(q2).*sin(q3).*sin(q4))./2.0+cos(q1).*cos(q3).*cos(q4).*sin(q5).*sqrt(-sqrt(2.0)+2.0).*(3.0./4.0e+1)-cos(q2).*sin(q1).*sin(q4).*sin(q5).*sqrt(-sqrt(2.0)+2.0).*(3.0./4.0e+1)+(cos(q4).*sin(q1).*sin(q2).*sin(q3).*sin(q5))./1.0e+1-cos(q2).*cos(q4).*sin(q1).*sin(q6).*sqrt(sqrt(2.0)+2.0).*(3.0./4.0e+1);
    et38 = cos(q1).*cos(q3).*sin(q4).*sin(q6).*sqrt(sqrt(2.0)+2.0).*(-3.0./4.0e+1)+cos(q4).*sin(q1).*sin(q2).*sin(q3).*sin(q5).*sqrt(-sqrt(2.0)+2.0).*(3.0./4.0e+1)+cos(q1).*cos(q3).*cos(q4).*cos(q5).*cos(q6).*sqrt(sqrt(2.0)+2.0).*(3.0./4.0e+1)-cos(q2).*cos(q5).*cos(q6).*sin(q1).*sin(q4).*sqrt(sqrt(2.0)+2.0).*(3.0./4.0e+1)-sin(q1).*sin(q2).*sin(q3).*sin(q4).*sin(q6).*sqrt(sqrt(2.0)+2.0).*(3.0./4.0e+1)+cos(q4).*cos(q5).*cos(q6).*sin(q1).*sin(q2).*sin(q3).*sqrt(sqrt(2.0)+2.0).*(3.0./4.0e+1);
    et39 = (sin(q1).*sin(q3).*sin(q5))./1.0e+1+sin(q1).*sin(q3).*sin(q5).*sqrt(-sqrt(2.0)+2.0).*(3.0./4.0e+1)-(cos(q1).*cos(q2).*cos(q4).*cos(q5))./1.0e+1+(cos(q1).*cos(q3).*sin(q2).*sin(q5))./1.0e+1+(cos(q3).*cos(q5).*sin(q1).*sin(q4))./1.0e+1-cos(q1).*cos(q2).*cos(q4).*cos(q5).*sqrt(-sqrt(2.0)+2.0).*(3.0./4.0e+1)+cos(q1).*cos(q3).*sin(q2).*sin(q5).*sqrt(-sqrt(2.0)+2.0).*(3.0./4.0e+1)+cos(q3).*cos(q5).*sin(q1).*sin(q4).*sqrt(-sqrt(2.0)+2.0).*(3.0./4.0e+1)-(cos(q1).*cos(q5).*sin(q2).*sin(q3).*sin(q4))./1.0e+1+cos(q5).*cos(q6).*sin(q1).*sin(q3).*sqrt(sqrt(2.0)+2.0).*(3.0./4.0e+1);
    et40 = cos(q1).*cos(q5).*sin(q2).*sin(q3).*sin(q4).*sqrt(-sqrt(2.0)+2.0).*(-3.0./4.0e+1)+cos(q1).*cos(q3).*cos(q5).*cos(q6).*sin(q2).*sqrt(sqrt(2.0)+2.0).*(3.0./4.0e+1)+cos(q1).*cos(q2).*cos(q4).*cos(q6).*sin(q5).*sqrt(sqrt(2.0)+2.0).*(3.0./4.0e+1)-cos(q3).*cos(q6).*sin(q1).*sin(q4).*sin(q5).*sqrt(sqrt(2.0)+2.0).*(3.0./4.0e+1)+cos(q1).*cos(q6).*sin(q2).*sin(q3).*sin(q4).*sin(q5).*sqrt(sqrt(2.0)+2.0).*(3.0./4.0e+1);
    et41 = (cos(q1).*sin(q3).*sin(q5))./1.0e+1+cos(q1).*sin(q3).*sin(q5).*sqrt(-sqrt(2.0)+2.0).*(3.0./4.0e+1)+(cos(q2).*cos(q4).*cos(q5).*sin(q1))./1.0e+1+(cos(q1).*cos(q3).*cos(q5).*sin(q4))./1.0e+1-(cos(q3).*sin(q1).*sin(q2).*sin(q5))./1.0e+1+cos(q2).*cos(q4).*cos(q5).*sin(q1).*sqrt(-sqrt(2.0)+2.0).*(3.0./4.0e+1)+cos(q1).*cos(q3).*cos(q5).*sin(q4).*sqrt(-sqrt(2.0)+2.0).*(3.0./4.0e+1)-cos(q3).*sin(q1).*sin(q2).*sin(q5).*sqrt(-sqrt(2.0)+2.0).*(3.0./4.0e+1)+(cos(q5).*sin(q1).*sin(q2).*sin(q3).*sin(q4))./1.0e+1+cos(q1).*cos(q5).*cos(q6).*sin(q3).*sqrt(sqrt(2.0)+2.0).*(3.0./4.0e+1);
    et42 = cos(q5).*sin(q1).*sin(q2).*sin(q3).*sin(q4).*sqrt(-sqrt(2.0)+2.0).*(3.0./4.0e+1)-cos(q3).*cos(q5).*cos(q6).*sin(q1).*sin(q2).*sqrt(sqrt(2.0)+2.0).*(3.0./4.0e+1)-cos(q2).*cos(q4).*cos(q6).*sin(q1).*sin(q5).*sqrt(sqrt(2.0)+2.0).*(3.0./4.0e+1)-cos(q1).*cos(q3).*cos(q6).*sin(q4).*sin(q5).*sqrt(sqrt(2.0)+2.0).*(3.0./4.0e+1)-cos(q6).*sin(q1).*sin(q2).*sin(q3).*sin(q4).*sin(q5).*sqrt(sqrt(2.0)+2.0).*(3.0./4.0e+1);
    et43 = sin(q1).*sin(q3).*sin(q5).*sin(q6).*sqrt(sqrt(2.0)+2.0).*(-3.0./4.0e+1)+cos(q1).*cos(q2).*cos(q6).*sin(q4).*sqrt(sqrt(2.0)+2.0).*(3.0./4.0e+1)+cos(q3).*cos(q4).*cos(q6).*sin(q1).*sqrt(sqrt(2.0)+2.0).*(3.0./4.0e+1)+cos(q1).*cos(q2).*cos(q4).*cos(q5).*sin(q6).*sqrt(sqrt(2.0)+2.0).*(3.0./4.0e+1)-cos(q1).*cos(q4).*cos(q6).*sin(q2).*sin(q3).*sqrt(sqrt(2.0)+2.0).*(3.0./4.0e+1)-cos(q1).*cos(q3).*sin(q2).*sin(q5).*sin(q6).*sqrt(sqrt(2.0)+2.0).*(3.0./4.0e+1)-cos(q3).*cos(q5).*sin(q1).*sin(q4).*sin(q6).*sqrt(sqrt(2.0)+2.0).*(3.0./4.0e+1);
    et44 = cos(q1).*cos(q5).*sin(q2).*sin(q3).*sin(q4).*sin(q6).*sqrt(sqrt(2.0)+2.0).*(3.0./4.0e+1);
    et45 = cos(q1).*cos(q3).*cos(q4).*cos(q6).*sqrt(sqrt(2.0)+2.0).*(3.0./4.0e+1)-cos(q2).*cos(q6).*sin(q1).*sin(q4).*sqrt(sqrt(2.0)+2.0).*(3.0./4.0e+1)-cos(q1).*sin(q3).*sin(q5).*sin(q6).*sqrt(sqrt(2.0)+2.0).*(3.0./4.0e+1)-cos(q2).*cos(q4).*cos(q5).*sin(q1).*sin(q6).*sqrt(sqrt(2.0)+2.0).*(3.0./4.0e+1)-cos(q1).*cos(q3).*cos(q5).*sin(q4).*sin(q6).*sqrt(sqrt(2.0)+2.0).*(3.0./4.0e+1)+cos(q4).*cos(q6).*sin(q1).*sin(q2).*sin(q3).*sqrt(sqrt(2.0)+2.0).*(3.0./4.0e+1)+cos(q3).*sin(q1).*sin(q2).*sin(q5).*sin(q6).*sqrt(sqrt(2.0)+2.0).*(3.0./4.0e+1);
    et46 = cos(q5).*sin(q1).*sin(q2).*sin(q3).*sin(q4).*sin(q6).*sqrt(sqrt(2.0)+2.0).*(-3.0./4.0e+1);
    mt5 = [et20+et21+et22,et17+et18+et19,0.0,0.0,0.0,1.0,(sin(q1).*(et27+et28))./4.0e+1,cos(q1).*(et25+et26).*(-1.0./4.0e+1),et23+et24,cos(q1),sin(q1),0.0,et31+et32,et29+et30,(cos(q2).*(cos(q3).*cos(q4).*2.0e+1-cos(q3).*sin(q4).*4.0-cos(q5).*sin(q3).*4.0-cos(q5).*sin(q3).*sqrt(-sqrt(2.0)+2.0).*3.0+cos(q3).*sin(q4).*sin(q5).*4.0+cos(q3).*cos(q4).*sin(q6).*sqrt(sqrt(2.0)+2.0).*3.0+cos(q6).*sin(q3).*sin(q5).*sqrt(sqrt(2.0)+2.0).*3.0+cos(q3).*sin(q4).*sin(q5).*sqrt(-sqrt(2.0)+2.0).*3.0+cos(q3).*cos(q5).*cos(q6).*sin(q4).*sqrt(sqrt(2.0)+2.0).*3.0))./4.0e+1,cos(q2).*sin(q1),-cos(q1).*cos(q2)];
    mt6 = [-sin(q2),et37+et38,et35+et36,et33+et34,-cos(q1).*sin(q3)+cos(q3).*sin(q1).*sin(q2),-sin(q1).*sin(q3)-cos(q1).*cos(q3).*sin(q2),cos(q2).*cos(q3),et41+et42,et39+et40];
    mt7 = [cos(q2).*cos(q3).*sin(q5).*(-1.0./1.0e+1)-(cos(q4).*cos(q5).*sin(q2))./1.0e+1-cos(q2).*cos(q3).*sin(q5).*sqrt(-sqrt(2.0)+2.0).*(3.0./4.0e+1)-cos(q4).*cos(q5).*sin(q2).*sqrt(-sqrt(2.0)+2.0).*(3.0./4.0e+1)+(cos(q2).*cos(q5).*sin(q3).*sin(q4))./1.0e+1+cos(q2).*cos(q5).*sin(q3).*sin(q4).*sqrt(-sqrt(2.0)+2.0).*(3.0./4.0e+1)-cos(q2).*cos(q3).*cos(q5).*cos(q6).*sqrt(sqrt(2.0)+2.0).*(3.0./4.0e+1)+cos(q4).*cos(q6).*sin(q2).*sin(q5).*sqrt(sqrt(2.0)+2.0).*(3.0./4.0e+1)-cos(q2).*cos(q6).*sin(q3).*sin(q4).*sin(q5).*sqrt(sqrt(2.0)+2.0).*(3.0./4.0e+1)];
    mt8 = [cos(q1).*cos(q3).*cos(q4)-cos(q2).*sin(q1).*sin(q4)+cos(q4).*sin(q1).*sin(q2).*sin(q3),cos(q1).*cos(q2).*sin(q4)+cos(q3).*cos(q4).*sin(q1)-cos(q1).*cos(q4).*sin(q2).*sin(q3),sin(q2).*sin(q4)+cos(q2).*cos(q4).*sin(q3),et45+et46,et43+et44,cos(q6).*sin(q2).*sin(q4).*sqrt(sqrt(2.0)+2.0).*(3.0./4.0e+1)+cos(q2).*cos(q4).*cos(q6).*sin(q3).*sqrt(sqrt(2.0)+2.0).*(3.0./4.0e+1)+cos(q2).*cos(q3).*sin(q5).*sin(q6).*sqrt(sqrt(2.0)+2.0).*(3.0./4.0e+1)+cos(q4).*cos(q5).*sin(q2).*sin(q6).*sqrt(sqrt(2.0)+2.0).*(3.0./4.0e+1)-cos(q2).*cos(q5).*sin(q3).*sin(q4).*sin(q6).*sqrt(sqrt(2.0)+2.0).*(3.0./4.0e+1)];
    mt9 = [-cos(q1).*cos(q5).*sin(q3)+cos(q3).*cos(q5).*sin(q1).*sin(q2)+cos(q2).*cos(q4).*sin(q1).*sin(q5)+cos(q1).*cos(q3).*sin(q4).*sin(q5)+sin(q1).*sin(q2).*sin(q3).*sin(q4).*sin(q5),-cos(q5).*sin(q1).*sin(q3)-cos(q1).*cos(q3).*cos(q5).*sin(q2)-cos(q1).*cos(q2).*cos(q4).*sin(q5)+cos(q3).*sin(q1).*sin(q4).*sin(q5)-cos(q1).*sin(q2).*sin(q3).*sin(q4).*sin(q5),cos(q2).*cos(q3).*cos(q5)-cos(q4).*sin(q2).*sin(q5)+cos(q2).*sin(q3).*sin(q4).*sin(q5)];
    J = reshape([mt5,mt6,mt7,mt8,mt9],6,6);
end
end
